simulink model "IMU"  (R2023b)
settings: Solver=VariableStepAuto  StartTime=0.0  StopTime=10.0  RelTol=1e-3
settings Model: Creator=lucaerviati  LastModifiedBy=carol
settings OptimizationCC: ReuseModelBlockBuffer=off

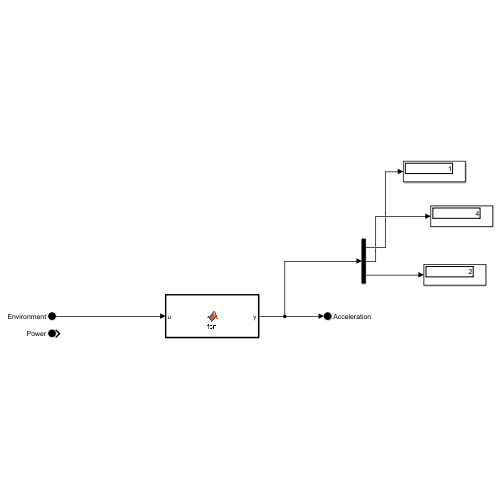
[thumbnail: Simulink's stored preview of the top-level diagram]
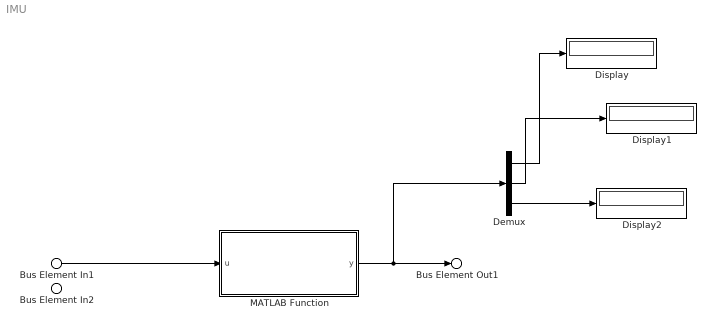
== system IMU ==
  Bus Element In1 : Inport  PortName=Environment
  Bus Element In2 : Inport  Port=2  PortName=Power
  Demux : Demux  Outputs=3
  Display : Display
  Display1 : Display
  Display2 : Display
  MATLAB Function : MATLAB Function  TreatAsAtomicUnit=on
  Bus Element Out1 : Outport  PortName=Acceleration
  wires:
  MATLAB Function/1(y) -> Demux/1, Bus Element Out1/1
  Bus Element In1/1 -> MATLAB Function/1(u)
  Demux/1 -> Display/1
  Demux/3 -> Display2/1
  Demux/2 -> Display1/1

== matlab function IMU/MATLAB Function ==
  data: u input; y output
function y = fcn(u)
u = [001,
    004,
    2]
y = u;
